simulink model "faultHandling_combined"  (R2018a)
settings: Solver=VariableStepAuto  StartTime=0.0  StopTime=100  FixedStep=1e-2  MaxStep=1e-1  MinStep=1e-6  RelTol=1e-9
undefined symbols (not defined in the file): b, I, I_wheel, K, k_e, k_t, kd, ki, kp, L, magnitude, R
libraries: aausat3_lib x30, dspindex x3, sharedutil x1, library x1
(part 2 of 2)

== matlab function faultHandling_combined/TorqueControlledReactionWheel/Controlled Motor5/MATLAB Function1 ==
  data: omega input; out output; time input; b input
function out = fcn(omega, time, b)

out = omega*b;

% if(time > 30)
%    out = 2*omega*b;
% end

== matlab function faultHandling_combined/TorqueControlledReactionWheel/Omega Control2/MATLAB Function1 ==
  data: omega input; out output; time input; b input
function out = fcn(omega, time, b)

out = omega*b;

% if(time > 30)
%    out = 2*omega*b;
% end

== matlab function faultHandling_combined/TorqueControlledReactionWheel/Controlled Motor6/MATLAB Function1 ==
  data: omega input; out output; time input; b input
function out = fcn(omega, time, b)

out = omega*b;

% if(time > 30)
%    out = 2*omega*b;
% end

== matlab function faultHandling_combined/TorqueControlledReactionWheel/Omega Control3/MATLAB Function1 ==
  data: omega input; out output; time input; b input
function out = fcn(omega, time, b)

out = omega*b;

% if(time > 30)
%    out = 2*omega*b;
% end

== matlab function faultHandling_combined/TorqueControlledReactionWheel/ReactionWheel Supervisor System ==
  data: Residuals input; ReconfigurationSignal output; faultMemory input; residualFaultMemory input; residualFault output
function [ReconfigurationSignal, residualFault]   = fcn(Residuals, faultMemory, residualFaultMemory)

threshold = 1e-10; % adjustable threshold
% threshold = 10; % adjustable threshold
residualFault = residualFaultMemory;

error =  abs(Residuals) > threshold;

if(faultMemory == 0)
    if(error(1) == 1)
        ReconfigurationSignal = 1;
        residualFault = 1;
    elseif(error(2) == 1)
        ReconfigurationSignal = 2;
        residualFault = 1;
    elseif(error(3) == 1)
        ReconfigurationSignal = 3;
        residualFault = 1;
    elseif(error(4) == 1)
        ReconfigurationSignal = 4;
        residualFault = 1;
    else
        ReconfigurationSignal = 0;
    end
else
    ReconfigurationSignal = faultMemory;
end

== matlab function faultHandling_combined/Drag force based on orientation based on orbit and current orientation/MATLAB Function ==
  data: A input; u output
function u = fcn(A)

A_min = 0.01;
rapport = A/A_min;

u_min = 7.2700e-16;
u = u_min*rapport;

== matlab function faultHandling_combined/TorqueControlledReactionWheel/Controlled Motor7/TauOut Predictor/Output torque estimator ==
  data: i input; TauOut output; k_t input; b input; omega input
function TauOut   = fcn(i, k_t, b, omega)

TauOut = k_t*i - b*omega;

== matlab function faultHandling_combined/TorqueControlledReactionWheel/Controlled Motor8/MATLAB Function1 ==
  data: omega input; out output; time input; b input
function out = fcn(omega, time, b)

out = omega*b;

% if(time > 30)
%    out = 2*omega*b;
% end

== matlab function faultHandling_combined/TorqueControlledReactionWheel/Reaction wheel reconfiguration ==
  data: reconfigSignal input; TorqueDemandWheel output; TauDemand input
function TorqueDemandWheel = fcn(reconfigSignal, TauDemand)


if(reconfigSignal == 1)
    
  TorqueDemandWheel =  [  0 0 0;
      0.6452    3.9841         0;
    0.6452   -3.9841         0;
    0.7503    0.0000    1.0000] * TauDemand;

elseif(reconfigSignal == 2)
    
  TorqueDemandWheel =  [     1.2291    7.5891         0;
      0 0 0;
         0   -7.9681         0;
    0.7146   -0.2204    1.0000] * TauDemand;
    
elseif(reconfigSignal == 3)
    
  TorqueDemandWheel =  [     1.2291   -7.5891   -0.0000;
    0.0000    7.9681    0.0000;
         0         0         0;
    0.7146    0.2204    1.0000] * TauDemand;
    
elseif(reconfigSignal == 4)
    
  TorqueDemandWheel =  [    25.8398    0.0000   34.4397;
  -12.9199    3.9841  -18.0799;
  -12.9199   -3.9841  -18.0799;
         0         0         0] * TauDemand;
    
else %(errorSignal == 0)
    
  TorqueDemandWheel = [0.4505   -0.0000    0.0187;
    0.4087    3.9840   -0.0098;
    0.4087   -3.9840   -0.0098;
    0.7372   -0.0000    0.9995] * TauDemand;
    
end

== matlab function faultHandling_combined/Disturbances/Computing JD ==
  data: t input; JD output
function JD = fcn(t)

JD0 = 2456293.520833 + 6*365;
sec_day = 60*60*24;

JD = JD0 + t/sec_day;
